simulink model "Spectrum_Analizer_2"  (R2020b)
settings: Solver=VariableStepAuto  StartTime=0.0  StopTime=100  RelTol=1e-3
InitFcn:
  | ts3=0.001;
  | dt=0.001;
libraries: dspsrcs4 x1, simulink x1
settings Model: Creator=TC16766  LastModifiedBy=TC16766

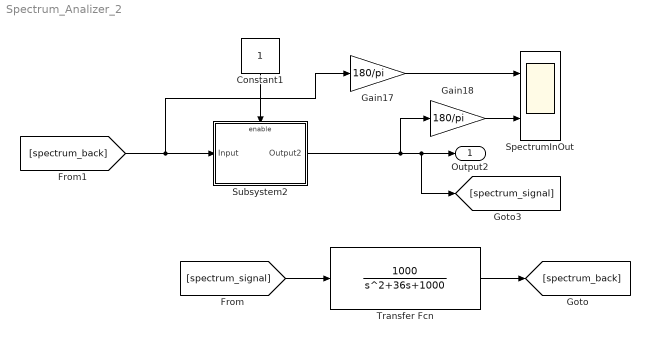
== system Spectrum_Analizer_2 ==
  Constant1 : Constant  OutDataTypeStr=boolean
      settings: AttributesFormatString=1 - START\n0 -STOP\ninternal spectrum
      settings: OpenFcn=|
      | if get_param(gcbh,'value')-48 set_param(gcbh,'value','0','backgroundcolor','red');
      | else set_param(gcbh,'value','1','backgroundcolor','green');
      | end
  Gain17 : Gain  Gain=180/pi
  Gain18 : Gain  Gain=180/pi
  SpectrumInOut : Scope  NumInputPorts=2
  Subsystem2 : Subsystem  mask{GAIN=1%2*pi/180%0.5*pi/180, InitFreq=1, TargetTime=100, FreqAtTime=100}
      mask prompts: InitFreq "INITIAL FREQUENCY"; TargetTime "Target Time"; FreqAtTime "Frequency at Time"
  Transfer Fcn : TransferFcn  Numerator=[1000]  Denominator=[1 36 1000]
  Output2 : Outport
  wires:
  Subsystem2/1(Output2) -> [spectrum_signal], Output2/1, Gain18/1
  Gain17/1 -> SpectrumInOut/1
  Gain18/1 -> SpectrumInOut/2
  [spectrum_back] -> Gain17/1, Subsystem2/1(Input)
  Constant1/1 -> Subsystem2/Enable
  [spectrum_signal] -> Transfer Fcn/1
  Transfer Fcn/1 -> [spectrum_back]

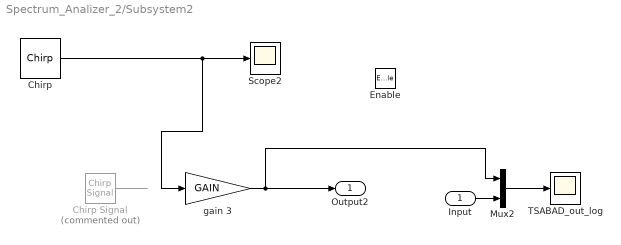
== system Spectrum_Analizer_2/Subsystem2 ==
  Input : Inport
  Enable : EnablePort  StatesWhenEnabling=reset
  Chirp : dspsrcs4/Chirp  sweep=Quadratic  mode=Unidirectional  f0=1  f1=FreqAtTime  t1=TargetTime  Tsweep=TargetTime  phase=0  Ts=1/1000  spf=1  datatype=Double  OutputFrames=off
  Chirp Signal : simulink/Sources/Chirp Signal  Commented=on  f1=InitFreq  T=TargetTime  f2=FreqAtTime
  Mux2 : Mux  Inputs=2
  Scope2 : Scope
  TSABAD_out_log : Scope
  gain 3 : Gain  Gain=GAIN  SaturateOnIntegerOverflow=on  SampleTime=ts3  OutDataTypeStr=Inherit: Same as input  ParamDataTypeStr=Inherit: Same as input
  Output2 : Outport
  wires:
  gain 3/1 -> Output2/1, Mux2/1
  Chirp Signal/1 -> ?
  Input/1 -> Mux2/2
  Mux2/1 -> TSABAD_out_log/1
  Chirp/1 -> gain 3/1, Scope2/1
